simulink model "scheme_1"  (R2017a)
settings: Solver=VariableStepAuto  StartTime=0.0  StopTime=25  RelTol=1e-3
libraries: simulink x1
settings Model: Creator=igorkislyuk  LastModifiedBy=igorkislyuk

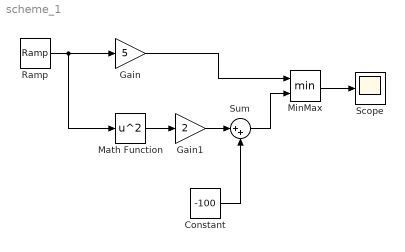
== system scheme_1 ==
  Constant : Constant  Value=-100
  Gain : Gain  Gain=5
  Gain1 : Gain  Gain=2
  Math Function : Math  Operator=square  SaturateOnIntegerOverflow=on
  MinMax : MinMax  Inputs=2
  Ramp : simulink/Sources/Ramp  slope=1  start=0  X0=0
  Scope : Scope
  Sum : Sum  Inputs=|++
  wires:
  Ramp/1 -> Math Function/1, Gain/1
  Gain/1 -> MinMax/1
  MinMax/1 -> Scope/1
  Math Function/1 -> Gain1/1
  Gain1/1 -> Sum/1
  Constant/1 -> Sum/2
  Sum/1 -> MinMax/2
